simulink library "FIN"  (R2016b)
settings: Solver=VariableStepAuto  StartTime=0.0  StopTime=10.0  RelTol=1e-3
undefined symbols (not defined in the file): AERO
libraries: aerolibutil x3, aerolibtransform2 x3, aerolibasang x2, simulink x2
settings Model: Creator=Andrew  LastModifiedBy=Andrew

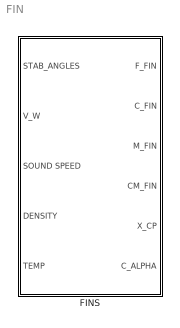
== system FIN ==
  FINS : Subsystem  mask{FIN=AERO.FIN(1)}
      mask prompts: FIN "FIN NUMBER"

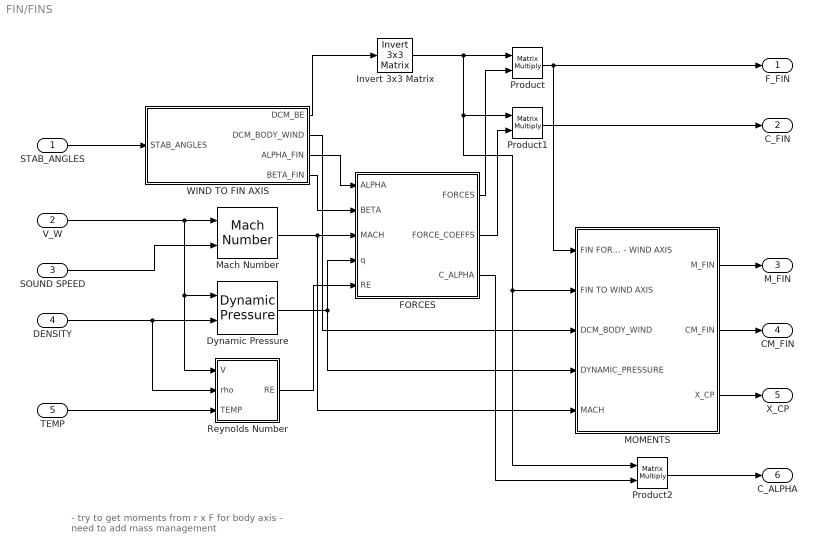
== system FIN/FINS ==
  note: - try to get moments from r x F for body axis
      | - need to add mass management
  STAB_ANGLES : Inport
  V_W : Inport  Port=2
  SOUND SPEED : Inport  Port=3
  DENSITY : Inport  Port=4
  TEMP : Inport  Port=5
  Dynamic Pressure : aerolibasang/Dynamic Pressure
  FORCES : Subsystem
  Invert 3x3 Matrix : aerolibutil/Invert  3x3 Matrix
  MOMENTS : Subsystem
  Mach Number : aerolibasang/Mach Number
  Product : Product  Multiplication=Matrix(*)
  Product1 : Product  Multiplication=Matrix(*)
  Product2 : Product  Multiplication=Matrix(*)
  Reynolds Number : Subsystem
  WIND TO FIN AXIS : Subsystem
  F_FIN : Outport
  C_FIN : Outport  Port=2
  M_FIN : Outport  Port=3
  CM_FIN : Outport  Port=4
  X_CP : Outport  Port=5
  C_ALPHA : Outport  Port=6
  wires:
  DENSITY/1 -> Reynolds Number/2(rho), Dynamic Pressure/2
  V_W/1 -> Reynolds Number/1(V), Dynamic Pressure/1, Mach Number/1
  SOUND SPEED/1 -> Mach Number/2
  Mach Number/1 -> MOMENTS/5(MACH), FORCES/3(MACH)
  Dynamic Pressure/1 -> MOMENTS/4(DYNAMIC_PRESSURE), FORCES/4(q)
  Product1/1 -> C_FIN/1
  WIND TO FIN AXIS/1(DCM_BE) -> Invert 3x3 Matrix/1
  FORCES/1(FORCES) -> Product/2
  FORCES/2(FORCE_COEFFS) -> Product1/2
  STAB_ANGLES/1 -> WIND TO FIN AXIS/1(STAB_ANGLES)
  TEMP/1 -> Reynolds Number/3(TEMP)
  WIND TO FIN AXIS/4(BETA_FIN) -> FORCES/2(BETA)
  WIND TO FIN AXIS/3(ALPHA_FIN) -> FORCES/1(ALPHA)
  Reynolds Number/1(RE) -> FORCES/5(RE)
  MOMENTS/2(CM_FIN) -> CM_FIN/1
  WIND TO FIN AXIS/2(DCM_BODY_WIND) -> MOMENTS/3(DCM_BODY_WIND)
  MOMENTS/1(M_FIN) -> M_FIN/1
  Invert 3x3 Matrix/1 -> MOMENTS/2(FIN TO WIND AXIS), Product2/1, Product1/1, Product/1
  Product/1 -> MOMENTS/1(FIN FORCES - WIND AXIS), F_FIN/1
  MOMENTS/3(X_CP) -> X_CP/1
  Product2/1 -> C_ALPHA/1
  FORCES/3(C_ALPHA) -> Product2/2

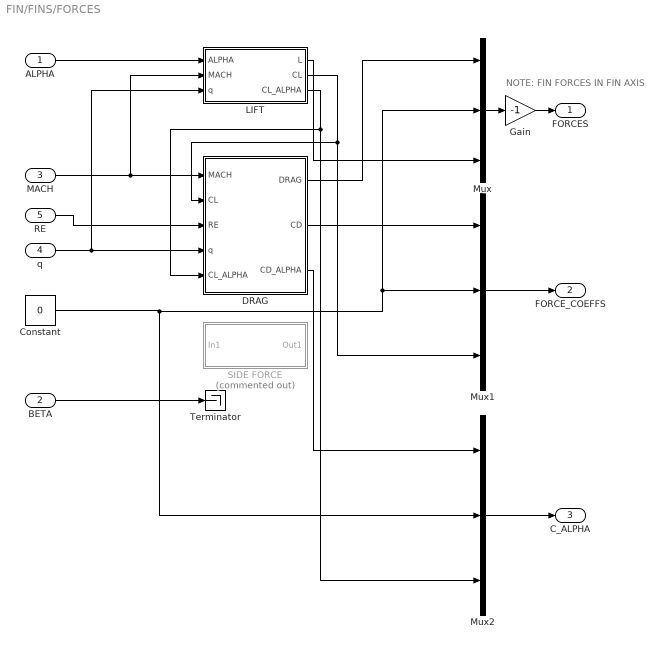
== system FIN/FINS/FORCES ==
  note: NOTE: FIN FORCES IN FIN AXIS
  ALPHA : Inport
  BETA : Inport  Port=2
  MACH : Inport  Port=3
  q : Inport  Port=4
  RE : Inport  Port=5
  Constant : Constant  Value=0
  DRAG : Subsystem
  Gain : Gain  Gain=-1
  LIFT : Subsystem
  Mux : Mux  Inputs=3
  Mux1 : Mux  Inputs=3
  Mux2 : Mux  Inputs=3
  SIDE FORCE : Subsystem  Commented=on
  Terminator : Terminator
  FORCES : Outport
  FORCE_COEFFS : Outport  Port=2
  C_ALPHA : Outport  Port=3
  wires:
  ALPHA/1 -> LIFT/1(ALPHA)
  Mux/1 -> Gain/1
  LIFT/1(L) -> Mux/3
  Mux1/1 -> FORCE_COEFFS/1
  LIFT/2(CL) -> Mux1/3, DRAG/2(CL)
  MACH/1 -> LIFT/2(MACH), DRAG/1(MACH)
  q/1 -> LIFT/3(q), DRAG/4(q)
  DRAG/1(DRAG) -> Mux/1
  DRAG/2(CD) -> Mux1/1
  RE/1 -> DRAG/3(RE)
  BETA/1 -> Terminator/1
  Gain/1 -> FORCES/1
  Constant/1 -> Mux2/2, Mux1/2, Mux/2
  LIFT/3(CL_ALPHA) -> Mux2/3, DRAG/5(CL_ALPHA)
  Mux2/1 -> C_ALPHA/1
  DRAG/3(CD_ALPHA) -> Mux2/1

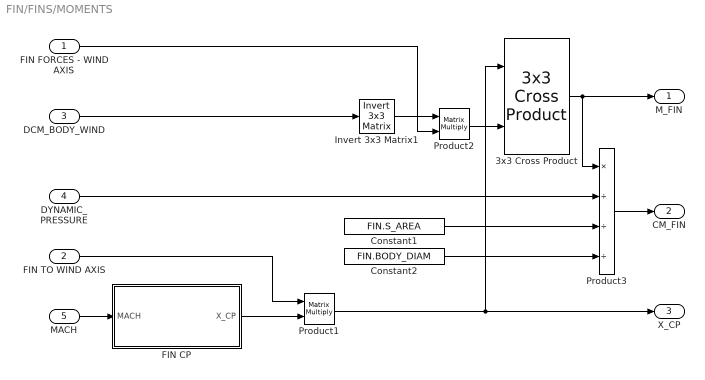
== system FIN/FINS/MOMENTS ==
  FIN FORCES - WIND AXIS : Inport
  FIN TO WIND AXIS : Inport  Port=2
  DCM_BODY_WIND : Inport  Port=3
  DYNAMIC_PRESSURE : Inport  Port=4
  MACH : Inport  Port=5
  3x3 Cross Product : aerolibutil/3x3 Cross Product
  Constant1 : Constant  Value=FIN.S_AREA
  Constant2 : Constant  Value=FIN.BODY_DIAM
  FIN CP : Subsystem
  Invert 3x3 Matrix1 : aerolibutil/Invert  3x3 Matrix
  Product1 : Product  Multiplication=Matrix(*)
  Product2 : Product  Multiplication=Matrix(*)
  Product3 : Product  Inputs=*///
  M_FIN : Outport
  CM_FIN : Outport  Port=2
  X_CP : Outport  Port=3
  wires:
  DCM_BODY_WIND/1 -> Invert 3x3 Matrix1/1
  Product2/1 -> 3x3 Cross Product/2
  Constant2/1 -> Product3/4
  3x3 Cross Product/1 -> M_FIN/1, Product3/1
  Invert 3x3 Matrix1/1 -> Product2/1
  Product3/1 -> CM_FIN/1
  Constant1/1 -> Product3/3
  DYNAMIC_PRESSURE/1 -> Product3/2
  FIN FORCES - WIND AXIS/1 -> Product2/2
  MACH/1 -> FIN CP/1(MACH)
  FIN CP/1(X_CP) -> Product1/2
  FIN TO WIND AXIS/1 -> Product1/1
  Product1/1 -> 3x3 Cross Product/1, X_CP/1

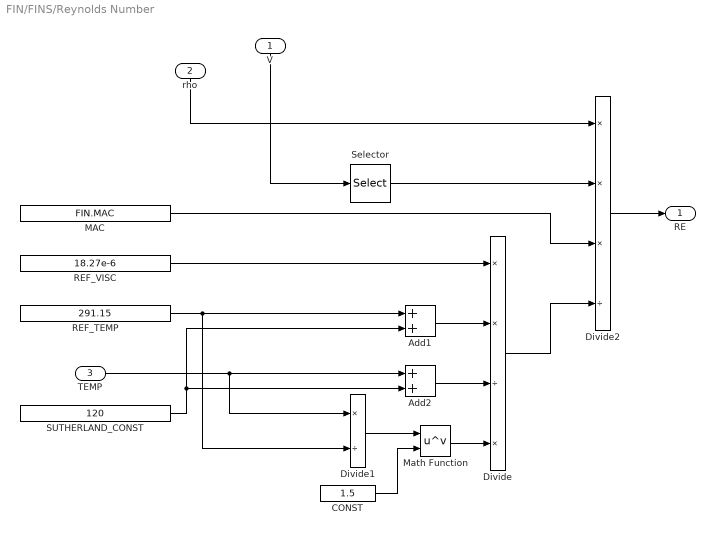
== system FIN/FINS/Reynolds Number ==
  V : Inport
  rho : Inport  Port=2
  TEMP : Inport  Port=3
  Add1 : Sum
  Add2 : Sum
  CONST : Constant  Value=1.5
  Divide : Product  Inputs=**/*
  Divide1 : Product  Inputs=*/
  Divide2 : Product  Inputs=***/
  MAC : Constant  Value=FIN.MAC
  Math Function : Math  Operator=pow  SaturateOnIntegerOverflow=on
  REF_TEMP : Constant  Value=291.15
  REF_VISC : Constant  Value=18.27e-6
  SUTHERLAND_CONST : Constant  Value=120
  Selector : Selector  InputPortWidth=3  IndexOptions=Index vector (dialog)  Indices=[1]  OutputSizes=1
  RE : Outport
  wires:
  Divide1/1 -> Math Function/1
  SUTHERLAND_CONST/1 -> Add1/2, Add2/2
  rho/1 -> Divide2/1
  V/1 -> Selector/1
  REF_TEMP/1 -> Add1/1, Divide1/2
  Divide2/1 -> RE/1
  REF_VISC/1 -> Divide/1
  Math Function/1 -> Divide/4
  Add1/1 -> Divide/2
  MAC/1 -> Divide2/3
  Add2/1 -> Divide/3
  CONST/1 -> Math Function/2
  TEMP/1 -> Divide1/1, Add2/1
  Divide/1 -> Divide2/4
  Selector/1 -> Divide2/2

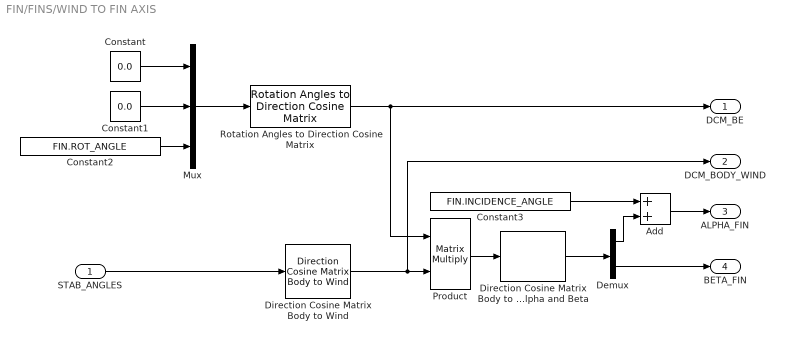
== system FIN/FINS/WIND TO FIN AXIS ==
  STAB_ANGLES : Inport
  Add : Sum
  Constant : Constant  Value=0.0
  Constant1 : Constant  Value=0.0
  Constant2 : Constant  Value=FIN.ROT_ANGLE
  Constant3 : Constant  Value=FIN.INCIDENCE_ANGLE
  Demux : Demux  Outputs=2
  Direction Cosine Matrix Body to Wind : aerolibtransform2/Direction Cosine Matrix Body to Wind
  Direction Cosine Matrix Body to Wind to Alpha and Beta : aerolibtransform2/Direction Cosine Matrix Body to Wind to Alpha and Beta
  Mux : Mux  Inputs=3
  Product : Product  Multiplication=Matrix(*)
  Rotation Angles to Direction Cosine Matrix : aerolibtransform2/Rotation Angles to Direction Cosine Matrix  rotationOrder=ZYX
  DCM_BE : Outport
  DCM_BODY_WIND : Outport  Port=2
  ALPHA_FIN : Outport  Port=3
  BETA_FIN : Outport  Port=4
  wires:
  Rotation Angles to Direction Cosine Matrix/1 -> Product/1, DCM_BE/1
  Demux/1 -> Add/2
  STAB_ANGLES/1 -> Direction Cosine Matrix Body to Wind/1
  Direction Cosine Matrix Body to Wind to Alpha and Beta/1 -> Demux/1
  Product/1 -> Direction Cosine Matrix Body to Wind to Alpha and Beta/1
  Constant1/1 -> Mux/2
  Add/1 -> ALPHA_FIN/1
  Mux/1 -> Rotation Angles to Direction Cosine Matrix/1
  Demux/2 -> BETA_FIN/1
  Constant/1 -> Mux/1
  Constant2/1 -> Mux/3
  Constant3/1 -> Add/1
  Direction Cosine Matrix Body to Wind/1 -> DCM_BODY_WIND/1, Product/2

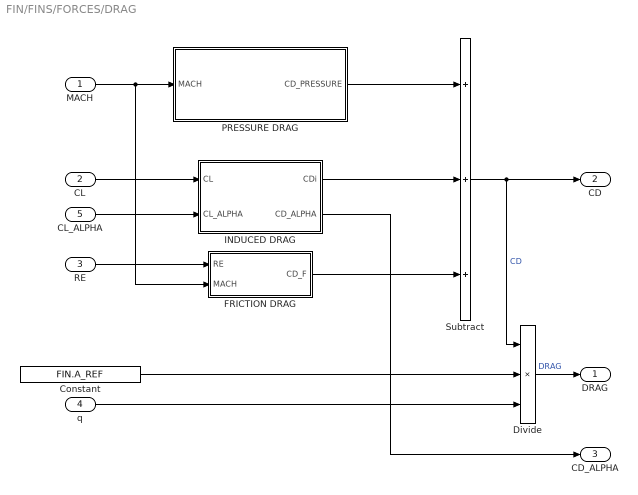
== system FIN/FINS/FORCES/DRAG ==
  MACH : Inport
  CL : Inport  Port=2
  RE : Inport  Port=3
  q : Inport  Port=4
  CL_ALPHA : Inport  Port=5
  Constant : Constant  Value=FIN.A_REF
  Divide : Product  Inputs=3
  FRICTION DRAG : Subsystem
  INDUCED DRAG : Subsystem
  PRESSURE DRAG : Subsystem
  Subtract : Sum  Inputs=+++
  DRAG : Outport
  CD : Outport  Port=2
  CD_ALPHA : Outport  Port=3
  wires:
  PRESSURE DRAG/1(CD_PRESSURE) -> Subtract/1
  Subtract/1 -> Divide/1, CD/1  "CD"
  Divide/1 -> DRAG/1  "DRAG"
  q/1 -> Divide/3
  Constant/1 -> Divide/2
  FRICTION DRAG/1(CD_F) -> Subtract/3
  INDUCED DRAG/1(CDi) -> Subtract/2
  CL/1 -> INDUCED DRAG/1(CL)
  RE/1 -> FRICTION DRAG/1(RE)
  MACH/1 -> FRICTION DRAG/2(MACH), PRESSURE DRAG/1(MACH)
  CL_ALPHA/1 -> INDUCED DRAG/2(CL_ALPHA)
  INDUCED DRAG/2(CD_ALPHA) -> CD_ALPHA/1

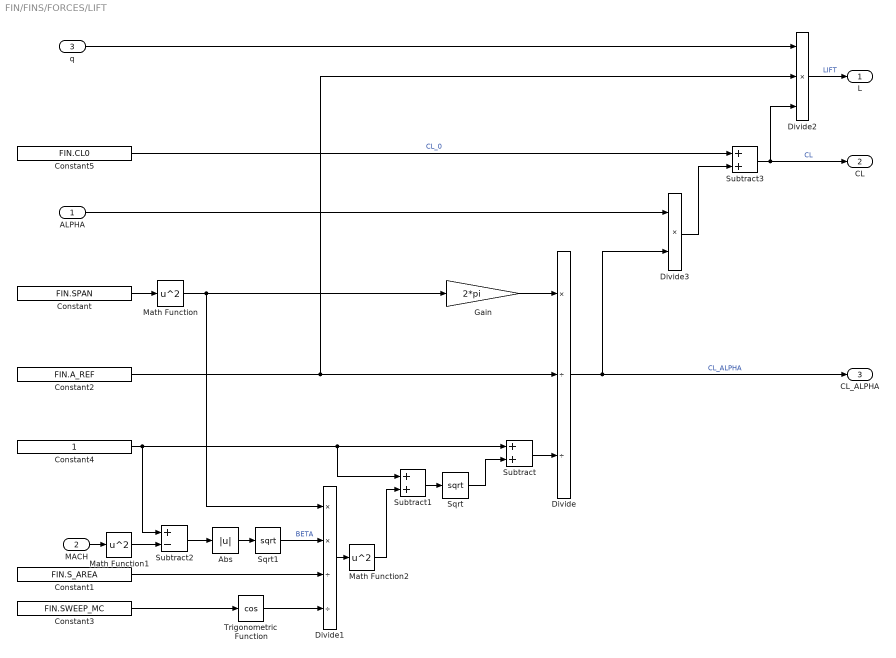
== system FIN/FINS/FORCES/LIFT ==
  ALPHA : Inport
  MACH : Inport  Port=2
  q : Inport  Port=3
  Abs : Abs
  Constant : Constant  Value=FIN.SPAN
  Constant1 : Constant  Value=FIN.S_AREA
  Constant2 : Constant  Value=FIN.A_REF
  Constant3 : Constant  Value=FIN.SWEEP_MC
  Constant4 : Constant
  Constant5 : Constant  Value=FIN.CL0  VectorParams1D=off
  Divide : Product  Inputs=*//
  Divide1 : Product  Inputs=**//
  Divide2 : Product  Inputs=***
  Divide3 : Product  Inputs=**
  Gain : Gain  Gain=2*pi
  Math Function : Math  Operator=square  SaturateOnIntegerOverflow=on
  Math Function1 : Math  Operator=square  SaturateOnIntegerOverflow=on
  Math Function2 : Math  Operator=square  SaturateOnIntegerOverflow=on
  Sqrt : Sqrt  SaturateOnIntegerOverflow=on
  Sqrt1 : Sqrt  SaturateOnIntegerOverflow=on
  Subtract : Sum
  Subtract1 : Sum
  Subtract2 : Sum  Inputs=+-
  Subtract3 : Sum
  Trigonometric Function : Trigonometry  Operator=cos
  L : Outport
  CL : Outport  Port=2
  CL_ALPHA : Outport  Port=3
  wires:
  Constant/1 -> Math Function/1
  Math Function/1 -> Divide1/1, Gain/1
  Constant4/1 -> Subtract1/1, Subtract/1, Subtract2/1
  Sqrt/1 -> Subtract/2
  Subtract1/1 -> Sqrt/1
  Constant1/1 -> Divide1/3
  Constant3/1 -> Trigonometric Function/1
  Trigonometric Function/1 -> Divide1/4
  MACH/1 -> Math Function1/1
  Abs/1 -> Sqrt1/1
  Divide1/1 -> Math Function2/1
  Math Function2/1 -> Subtract1/2
  Subtract2/1 -> Abs/1
  Math Function1/1 -> Subtract2/2
  Sqrt1/1 -> Divide1/2  "BETA"
  Subtract/1 -> Divide/3
  Constant2/1 -> Divide/2, Divide2/2
  Gain/1 -> Divide/1
  ALPHA/1 -> Divide3/1
  Constant5/1 -> Subtract3/1  "CL_0"
  Divide/1 -> CL_ALPHA/1, Divide3/2  "CL_ALPHA"
  Subtract3/1 -> CL/1, Divide2/3  "CL"
  Divide2/1 -> L/1  "LIFT"
  q/1 -> Divide2/1
  Divide3/1 -> Subtract3/2

== system FIN/FINS/FORCES/SIDE FORCE ==
  In1 : Inport
  Out1 : Outport
  wires:
  In1/1 -> Out1/1

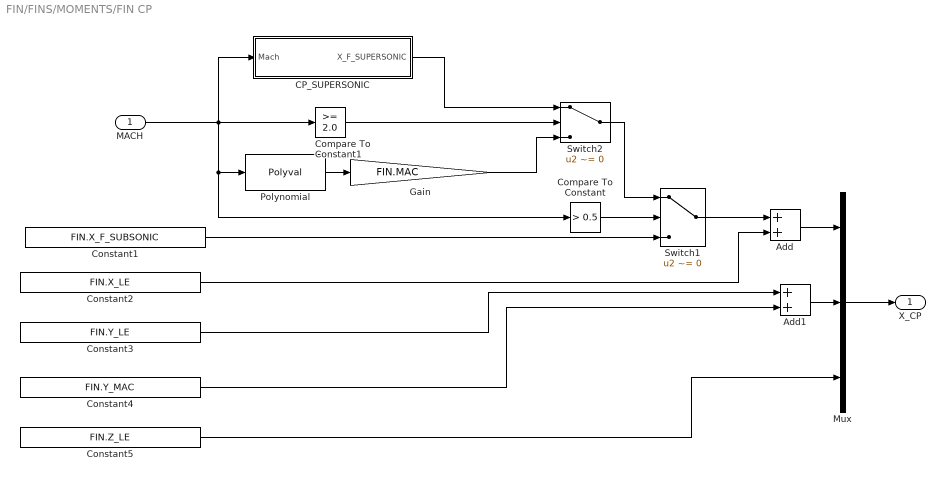
== system FIN/FINS/MOMENTS/FIN CP ==
  MACH : Inport
  Add : Sum
  Add1 : Sum
  CP_SUPERSONIC : Subsystem
  Compare To Constant : simulink/Logic and Bit Operations/Compare To Constant  relop=>  const=0.5  OutDataTypeStr=boolean
  Compare To Constant1 : simulink/Logic and Bit Operations/Compare To Constant  relop=>=  const=2.0  OutDataTypeStr=boolean
  Constant1 : Constant  Value=FIN.X_F_SUBSONIC
  Constant2 : Constant  Value=FIN.X_LE
  Constant3 : Constant  Value=FIN.Y_LE
  Constant4 : Constant  Value=FIN.Y_MAC
  Constant5 : Constant  Value=FIN.Z_LE
  Gain : Gain  Gain=FIN.MAC
  Mux : Mux  Inputs=3
  Polynomial : Polyval  Coefs=FIN.CP_COEFFS
  Switch1 : Switch  Criteria=u2 ~= 0
  Switch2 : Switch  Criteria=u2 ~= 0
  X_CP : Outport
  wires:
  MACH/1 -> Polynomial/1, Compare To Constant/1, CP_SUPERSONIC/1(Mach), Compare To Constant1/1
  CP_SUPERSONIC/1(X_F_SUPERSONIC) -> Switch2/1
  Switch2/1 -> Switch1/1
  Compare To Constant/1 -> Switch1/2
  Compare To Constant1/1 -> Switch2/2
  Constant1/1 -> Switch1/3
  Polynomial/1 -> Gain/1
  Gain/1 -> Switch2/3
  Mux/1 -> X_CP/1
  Add/1 -> Mux/1
  Switch1/1 -> Add/1
  Constant2/1 -> Add/2
  Add1/1 -> Mux/2
  Constant3/1 -> Add1/1
  Constant4/1 -> Add1/2
  Constant5/1 -> Mux/3

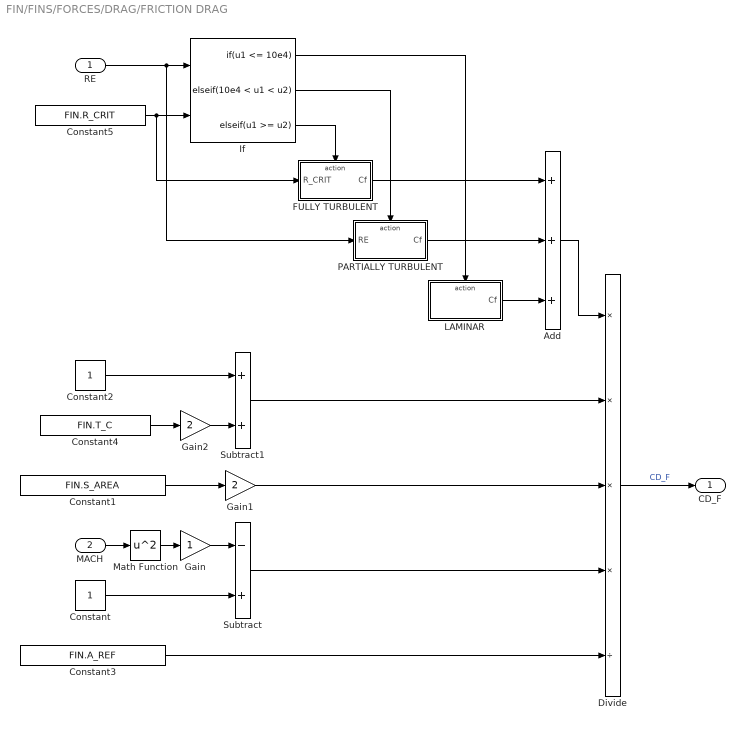
== system FIN/FINS/FORCES/DRAG/FRICTION DRAG ==
  RE : Inport
  MACH : Inport  Port=2
  Add : Sum  Inputs=+++
  Constant : Constant
  Constant1 : Constant  Value=FIN.S_AREA
  Constant2 : Constant
  Constant3 : Constant  Value=FIN.A_REF
  Constant4 : Constant  Value=FIN.T_C
  Constant5 : Constant  Value=FIN.R_CRIT
  Divide : Product  Inputs=****/
  FULLY TURBULENT : Subsystem  TreatAsAtomicUnit=on
  Gain : Gain
  Gain1 : Gain  Gain=2
  Gain2 : Gain  Gain=2
  If : If  NumInputs=2  IfExpression=u1 <= 10e4  ElseIfExpressions=10e4 < u1 < u2, u1 >= u2  ShowElse=off
  LAMINAR : Subsystem  TreatAsAtomicUnit=on
  Math Function : Math  Operator=square  SaturateOnIntegerOverflow=on
  PARTIALLY TURBULENT : Subsystem  TreatAsAtomicUnit=on
  Subtract : Sum  Inputs=-+
  Subtract1 : Sum
  CD_F : Outport
  wires:
  Divide/1 -> CD_F/1  "CD_F"
  MACH/1 -> Math Function/1
  Math Function/1 -> Gain/1
  Gain/1 -> Subtract/1
  Constant/1 -> Subtract/2
  Subtract/1 -> Divide/4
  Constant1/1 -> Gain1/1
  Gain1/1 -> Divide/3
  Subtract1/1 -> Divide/2
  Constant2/1 -> Subtract1/1
  Constant4/1 -> Gain2/1
  Gain2/1 -> Subtract1/2
  Constant3/1 -> Divide/5
  If/3 -> FULLY TURBULENT/Action
  If/2 -> PARTIALLY TURBULENT/Action
  If/1 -> LAMINAR/Action
  Constant5/1 -> FULLY TURBULENT/1(R_CRIT), If/2
  Add/1 -> Divide/1
  FULLY TURBULENT/1(Cf) -> Add/1
  LAMINAR/1(Cf) -> Add/3
  PARTIALLY TURBULENT/1(Cf) -> Add/2
  RE/1 -> PARTIALLY TURBULENT/1(RE), If/1

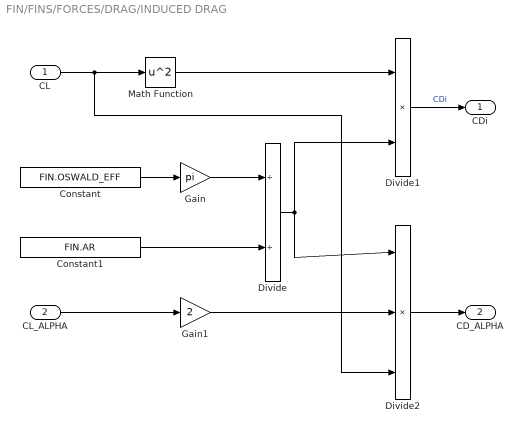
== system FIN/FINS/FORCES/DRAG/INDUCED DRAG ==
  CL : Inport
  CL_ALPHA : Inport  Port=2
  Constant : Constant  Value=FIN.OSWALD_EFF
  Constant1 : Constant  Value=FIN.AR
  Divide : Product  Inputs=//
  Divide1 : Product  Inputs=**
  Divide2 : Product  Inputs=***
  Gain : Gain  Gain=pi
  Gain1 : Gain  Gain=2
  Math Function : Math  Operator=square  SaturateOnIntegerOverflow=on
  CDi : Outport
  CD_ALPHA : Outport  Port=2
  wires:
  Constant/1 -> Gain/1
  Constant1/1 -> Divide/2
  Gain/1 -> Divide/1
  CL/1 -> Divide2/3, Math Function/1
  Math Function/1 -> Divide1/1
  Divide1/1 -> CDi/1  "CDi"
  Divide2/1 -> CD_ALPHA/1
  Divide/1 -> Divide2/1, Divide1/2
  CL_ALPHA/1 -> Gain1/1
  Gain1/1 -> Divide2/2

== system FIN/FINS/FORCES/DRAG/PRESSURE DRAG ==
  MACH : Inport
  Add : Sum
  Leading Edge : Subsystem
  Trailing Edge : Subsystem
  CD_PRESSURE : Outport
  wires:
  Add/1 -> CD_PRESSURE/1
  Leading Edge/1(CD_FIN_LE) -> Add/1
  MACH/1 -> Trailing Edge/1(MACH), Leading Edge/1(MACH)
  Trailing Edge/1(CD_FIN_TE) -> Add/2

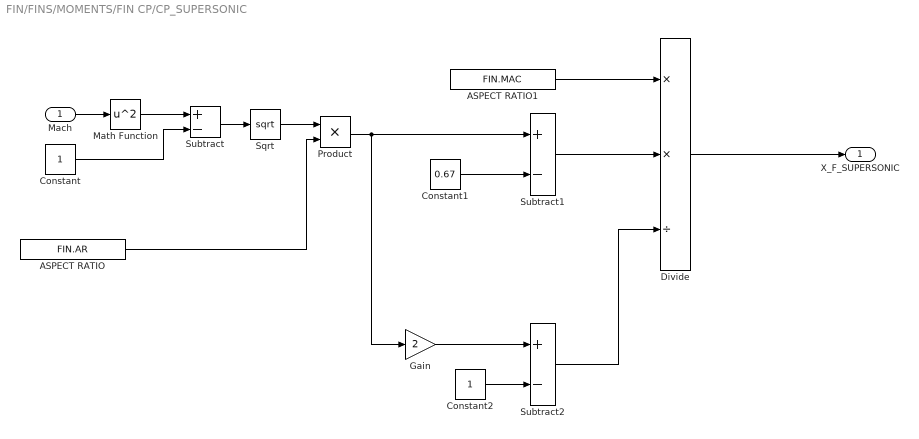
== system FIN/FINS/MOMENTS/FIN CP/CP_SUPERSONIC ==
  Mach : Inport
  ASPECT RATIO : Constant  Value=FIN.AR
  ASPECT RATIO1 : Constant  Value=FIN.MAC
  Constant : Constant
  Constant1 : Constant  Value=0.67
  Constant2 : Constant
  Divide : Product  Inputs=**/
  Gain : Gain  Gain=2
  Math Function : Math  Operator=square  SaturateOnIntegerOverflow=on
  Product : Product
  Sqrt : Sqrt  SaturateOnIntegerOverflow=on
  Subtract : Sum  Inputs=+-
  Subtract1 : Sum  Inputs=+-
  Subtract2 : Sum  Inputs=+-
  X_F_SUPERSONIC : Outport
  wires:
  Mach/1 -> Math Function/1
  Constant/1 -> Subtract/2
  Math Function/1 -> Subtract/1
  Subtract/1 -> Sqrt/1
  Sqrt/1 -> Product/1
  ASPECT RATIO/1 -> Product/2
  Product/1 -> Gain/1, Subtract1/1
  Constant1/1 -> Subtract1/2
  Constant2/1 -> Subtract2/2
  Subtract1/1 -> Divide/2
  Subtract2/1 -> Divide/3
  Divide/1 -> X_F_SUPERSONIC/1
  Gain/1 -> Subtract2/1
  ASPECT RATIO1/1 -> Divide/1

== system FIN/FINS/FORCES/DRAG/FRICTION DRAG/FULLY TURBULENT ==
  R_CRIT : Inport
  Action Port : ActionPort  ActionType=elseif
  Constant : Constant  Value=0.2/(-1.039)
  Gain : Gain  Gain=1/51
  Gain1 : Gain  Gain=0.032
  Math Function : Math  Operator=pow  SaturateOnIntegerOverflow=on
  Cf : Outport
  wires:
  R_CRIT/1 -> Gain/1
  Gain/1 -> Math Function/1
  Constant/1 -> Math Function/2
  Math Function/1 -> Gain1/1
  Gain1/1 -> Cf/1

== system FIN/FINS/FORCES/DRAG/FRICTION DRAG/LAMINAR ==
  Action Port : ActionPort  ActionType=then
  Constant : Constant  Value=1.48e-2
  Cf : Outport
  wires:
  Constant/1 -> Cf/1

== system FIN/FINS/FORCES/DRAG/FRICTION DRAG/PARTIALLY TURBULENT ==
  RE : Inport
  Action Port : ActionPort  ActionType=elseif
  Constant : Constant
  Constant1 : Constant  Value=5.6
  Divide : Product  Inputs=*/
  Gain : Gain  Gain=1.50
  Math Function : Math  Operator=log  SaturateOnIntegerOverflow=on
  Math Function1 : Math  Operator=square  SaturateOnIntegerOverflow=on
  Subtract : Sum  Inputs=+-
  Cf : Outport
  wires:
  Constant/1 -> Divide/1
  Divide/1 -> Cf/1
  RE/1 -> Math Function/1
  Gain/1 -> Subtract/1
  Math Function/1 -> Gain/1
  Subtract/1 -> Math Function1/1
  Math Function1/1 -> Divide/2
  Constant1/1 -> Subtract/2

== system FIN/FINS/FORCES/DRAG/PRESSURE DRAG/Leading Edge ==
  MACH : Inport
  Constant : Constant  Value=FIN.ROUNDED_LEADING_EDGE
  Constant1 : Constant  Value=FIN.SWEEP
  Constant2 : Constant  Value=FIN.SPAN
  Divide : Product  Inputs=**
  Divide1 : Product  Inputs=*/
  Rectangular Leading Edge : Subsystem
  Rounded Leading Edge : Subsystem
  Switch : Switch  Criteria=u2 ~= 0
  Trigonometric Function : Trigonometry  Operator=atan
  CD_FIN_LE : Outport
  wires:
  Divide/1 -> CD_FIN_LE/1
  MACH/1 -> Rectangular Leading Edge/1(MACH), Rounded Leading Edge/1(MACH)
  Divide1/1 -> Trigonometric Function/1
  Trigonometric Function/1 -> Divide/2
  Switch/1 -> Divide/1
  Constant1/1 -> Divide1/1
  Constant2/1 -> Divide1/2
  Constant/1 -> Switch/2
  Rectangular Leading Edge/1(CD_FIN_LE) -> Switch/3
  Rounded Leading Edge/1(CD_FIN_LE) -> Switch/1

== system FIN/FINS/FORCES/DRAG/PRESSURE DRAG/Trailing Edge ==
  MACH : Inport
  Add1 : Sum
  Constant : Constant  Value=FIN.ROUND_TRAIL_EDGE
  Constant1 : Constant  Value=FIN.TAPER_TRAIL_EDGE
  Constant2 : Constant  Value=0
  Gain : Gain  Gain=0.5
  If : If  IfExpression=u1<1
  Subsonic : Subsystem  TreatAsAtomicUnit=on
  Supersonic : Subsystem  TreatAsAtomicUnit=on
  Switch : Switch  Criteria=u2 ~= 0
  Switch1 : Switch  Criteria=u2 ~= 0
  CD_FIN_TE : Outport
  wires:
  Constant2/1 -> Switch1/1
  Constant1/1 -> Switch1/2
  Switch1/1 -> CD_FIN_TE/1
  Switch/1 -> Switch1/3
  Gain/1 -> Switch/1
  Constant/1 -> Switch/2
  Add1/1 -> Switch/3, Gain/1
  MACH/1 -> If/1, Subsonic/1(MACH), Supersonic/1(MACH)
  Supersonic/1(CD_FIN_LE) -> Add1/1
  Subsonic/1(CD_FIN_LE) -> Add1/2
  If/1 -> Subsonic/Action
  If/2 -> Supersonic/Action

== system FIN/FINS/FORCES/DRAG/PRESSURE DRAG/Leading Edge/Rectangular Leading Edge ==
  MACH : Inport
  Add1 : Sum
  If : If  IfExpression=u1<1
  Subsonic : Subsystem  TreatAsAtomicUnit=on
  Supersonic : Subsystem  TreatAsAtomicUnit=on
  CD_FIN_LE : Outport
  wires:
  Add1/1 -> CD_FIN_LE/1
  If/2 -> Supersonic/Action
  If/1 -> Subsonic/Action
  Subsonic/1(CD_FIN_LE) -> Add1/2
  Supersonic/1(CD_FIN_LE) -> Add1/1
  MACH/1 -> Supersonic/1(MACH), Subsonic/1(MACH), If/1

== system FIN/FINS/FORCES/DRAG/PRESSURE DRAG/Leading Edge/Rounded Leading Edge ==
  MACH : Inport
  Add1 : Sum  Inputs=+++
  If : If  IfExpression=u1<0.9  ElseIfExpressions=u1>1
  Subsonic : Subsystem  TreatAsAtomicUnit=on
  Supersonic : Subsystem  TreatAsAtomicUnit=on
  Transonic : Subsystem  TreatAsAtomicUnit=on
  CD_FIN_LE : Outport
  wires:
  MACH/1 -> If/1, Subsonic/1(MACH), Supersonic/1(MACH), Transonic/1(MACH)
  Supersonic/1(CD_FIN_LE) -> Add1/2
  Transonic/1(CD_FIN_LE) -> Add1/1
  Subsonic/1(CD_FIN_LE) -> Add1/3
  If/2 -> Supersonic/Action
  If/1 -> Subsonic/Action
  If/3 -> Transonic/Action
  Add1/1 -> CD_FIN_LE/1

== system FIN/FINS/FORCES/DRAG/PRESSURE DRAG/Trailing Edge/Subsonic ==
  note: CD_LE = 1 + M^2/4 + M^4 / 40
  MACH : Inport
  Action Port : ActionPort
  Constant : Constant  Value=0.12
  Gain : Gain  Gain=0.13
  Math Function : Math  Operator=square  SaturateOnIntegerOverflow=on
  Subtract : Sum
  CD_FIN_LE : Outport
  wires:
  Constant/1 -> Subtract/2
  Math Function/1 -> Gain/1
  MACH/1 -> Math Function/1
  Subtract/1 -> CD_FIN_LE/1
  Gain/1 -> Subtract/1

== system FIN/FINS/FORCES/DRAG/PRESSURE DRAG/Trailing Edge/Supersonic ==
  MACH : Inport
  Action Port : ActionPort
  Gain : Gain  Gain=0.25
  Math Function : Math  Operator=reciprocal  SaturateOnIntegerOverflow=on
  CD_FIN_LE : Outport
  wires:
  Gain/1 -> CD_FIN_LE/1
  MACH/1 -> Math Function/1
  Math Function/1 -> Gain/1

== system FIN/FINS/FORCES/DRAG/PRESSURE DRAG/Leading Edge/Rectangular Leading Edge/Subsonic ==
  note: CD_LE = 1 + M^2/4 + M^4 / 40
  MACH : Inport
  Action Port : ActionPort
  Constant : Constant
  Gain : Gain  Gain=0.25
  Gain1 : Gain  Gain=1/40
  Math Function : Math  Operator=square  SaturateOnIntegerOverflow=on
  Math Function1 : Math  Operator=square  SaturateOnIntegerOverflow=on
  Subtract : Sum  Inputs=+++
  CD_FIN_LE : Outport
  wires:
  Constant/1 -> Subtract/3
  Gain1/1 -> Subtract/2
  Math Function1/1 -> Gain1/1
  Gain/1 -> Subtract/1
  Subtract/1 -> CD_FIN_LE/1
  MACH/1 -> Math Function/1
  Math Function/1 -> Math Function1/1, Gain/1

== system FIN/FINS/FORCES/DRAG/PRESSURE DRAG/Leading Edge/Rectangular Leading Edge/Supersonic ==
  MACH : Inport
  Action Port : ActionPort
  Add : Sum  Inputs=+-++
  Constant : Constant  Value=1.84
  Gain : Gain  Gain=0.76
  Gain1 : Gain  Gain=0.166
  Gain2 : Gain  Gain=0.035
  Math Function : Math  Operator=reciprocal  SaturateOnIntegerOverflow=on
  Math Function1 : Math  Operator=square  SaturateOnIntegerOverflow=on
  Math Function2 : Math  Operator=square  SaturateOnIntegerOverflow=on
  Product : Product
  CD_FIN_LE : Outport
  wires:
  Gain2/1 -> Add/4
  Gain1/1 -> Add/3
  Product/1 -> Gain2/1
  Math Function1/1 -> Gain/1, Product/2, Math Function2/1
  Math Function2/1 -> Product/1, Gain1/1
  Math Function/1 -> Math Function1/1
  MACH/1 -> Math Function/1
  Add/1 -> CD_FIN_LE/1
  Constant/1 -> Add/1
  Gain/1 -> Add/2

== system FIN/FINS/FORCES/DRAG/PRESSURE DRAG/Leading Edge/Rounded Leading Edge/Subsonic ==
  note: CD_LE = (1 - M^2) ^(-0.417) - 1
  MACH : Inport
  Action Port : ActionPort
  Constant : Constant
  Constant1 : Constant  Value=-0.417
  Constant2 : Constant
  Math Function : Math  Operator=square  SaturateOnIntegerOverflow=on
  Math Function1 : Math  Operator=pow  SaturateOnIntegerOverflow=on
  Subtract : Sum  Inputs=+-
  Subtract1 : Sum  Inputs=+-
  CD_FIN_LE : Outport
  wires:
  Subtract1/1 -> CD_FIN_LE/1
  Constant2/1 -> Subtract1/2
  Math Function1/1 -> Subtract1/1
  Constant1/1 -> Math Function1/2
  Subtract/1 -> Math Function1/1
  Constant/1 -> Subtract/2
  Math Function/1 -> Subtract/1
  MACH/1 -> Math Function/1

== system FIN/FINS/FORCES/DRAG/PRESSURE DRAG/Leading Edge/Rounded Leading Edge/Supersonic ==
  MACH : Inport
  Action Port : ActionPort
  Add : Sum  Inputs=+-+
  Constant1 : Constant  Value=1.214
  Constant2 : Constant  Value=4
  Gain : Gain  Gain=0.502
  Gain1 : Gain  Gain=0.1095
  Math Function : Math  Operator=pow  SaturateOnIntegerOverflow=on
  Math Function1 : Math  Operator=square  SaturateOnIntegerOverflow=on
  Math Function2 : Math  Operator=reciprocal  SaturateOnIntegerOverflow=on
  CD_FIN_LE : Outport
  wires:
  Gain1/1 -> Add/1
  Math Function/1 -> Gain1/1
  Add/1 -> CD_FIN_LE/1
  Constant2/1 -> Math Function/2
  Gain/1 -> Add/2
  Math Function1/1 -> Gain/1
  Math Function2/1 -> Math Function/1, Math Function1/1
  MACH/1 -> Math Function2/1
  Constant1/1 -> Add/3

== system FIN/FINS/FORCES/DRAG/PRESSURE DRAG/Leading Edge/Rounded Leading Edge/Transonic ==
  MACH : Inport
  Action Port : ActionPort
  Add : Sum  Inputs=-+
  Add1 : Sum  Inputs=+-
  Constant : Constant
  Constant1 : Constant  Value=0.9
  Gain : Gain  Gain=1.785
  CD_FIN_LE : Outport
  wires:
  Gain/1 -> Add/2
  Add1/1 -> Gain/1
  Constant1/1 -> Add1/2
  MACH/1 -> Add1/1
  Constant/1 -> Add/1
  Add/1 -> CD_FIN_LE/1
